simulink model "linear_simulation"  (R2019b)
settings: Solver=VariableStepAuto  StartTime=0.0  StopTime=10.0  RelTol=1e-3
undefined symbols (not defined in the file or in its folder): k, Ki, Kp, omega_n, w, zeta
settings Model: Creator=jucat  LastModifiedBy=jucat

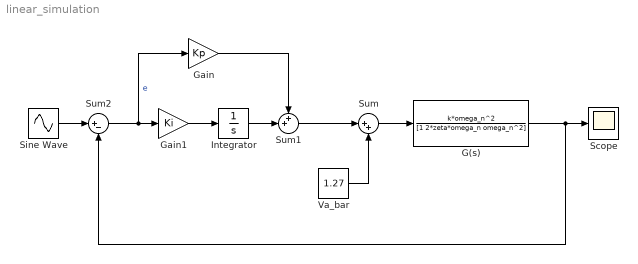
== system linear_simulation ==
  G(s) : TransferFcn  Numerator=k*omega_n^2  Denominator=[1 2*zeta*omega_n omega_n^2]
  Gain : Gain  Gain=Kp
  Gain1 : Gain  Gain=Ki
  Integrator : Integrator
  Scope : Scope
  Sine Wave : Sin  Amplitude=5  Bias=-30  Frequency=w  SampleTime=0
  Sum : Sum  Inputs=|++
  Sum1 : Sum  Inputs=++|
  Sum2 : Sum  Inputs=|+-
  Va_bar : Constant  Value=1.27
  wires:
  Sum/1 -> G(s)/1
  Va_bar/1 -> Sum/2
  Gain1/1 -> Integrator/1
  Integrator/1 -> Sum1/2
  Gain/1 -> Sum1/1
  Sum1/1 -> Sum/1
  G(s)/1 -> Sum2/2, Scope/1
  Sum2/1 -> Gain/1, Gain1/1  "e"
  Sine Wave/1 -> Sum2/1
